simulink model "teste_linearizacao"  (R2022a)
settings: Solver=VariableStepAuto  StartTime=0.0  StopTime=10.0  RelTol=1e-3
values from neighbouring files (symbols this model uses):
  C = [0 0 1 0]    [ball_and_beam_pfc.m]
  g = 9.8    [ball_and_beam_pfc.m]    (also in nonlinear_ball_and_beam.m)
  Jv = (1/2) * mv * L^2    (= 0.058703125)    [ball_and_beam_pfc.m]    (also in nonlinear_ball_and_beam.m)
  L = 0.425    [ball_and_beam_pfc.m]    (also in nonlinear_ball_and_beam.m)
  mb = 0.064    [ball_and_beam_pfc.m]    (also in nonlinear_ball_and_beam.m)
  mv = 0.65    [ball_and_beam_pfc.m]    (also in nonlinear_ball_and_beam.m)
settings Model: Creator=Notebook_Artur  LastModifiedBy=Notebook_Artur

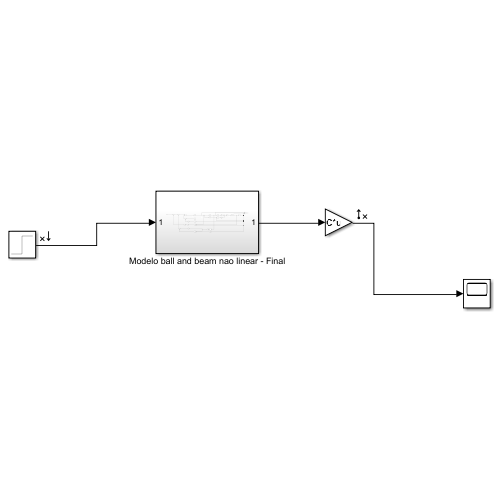
[thumbnail: Simulink's stored preview of the top-level diagram]
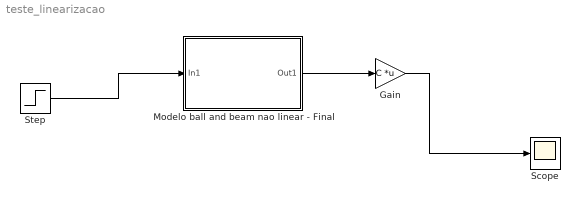
== system teste_linearizacao ==
  Gain : Gain  Gain=C  Multiplication=Matrix(K*u)
  Modelo ball and beam nao linear - Final : Subsystem
  Scope : Scope
  Step : Step  SampleTime=0
  wires:
  Step/1 -> Modelo ball and beam nao linear - Final/1(In1)
  Modelo ball and beam nao linear - Final/1(Out1) -> Gain/1
  Gain/1 -> Scope/1

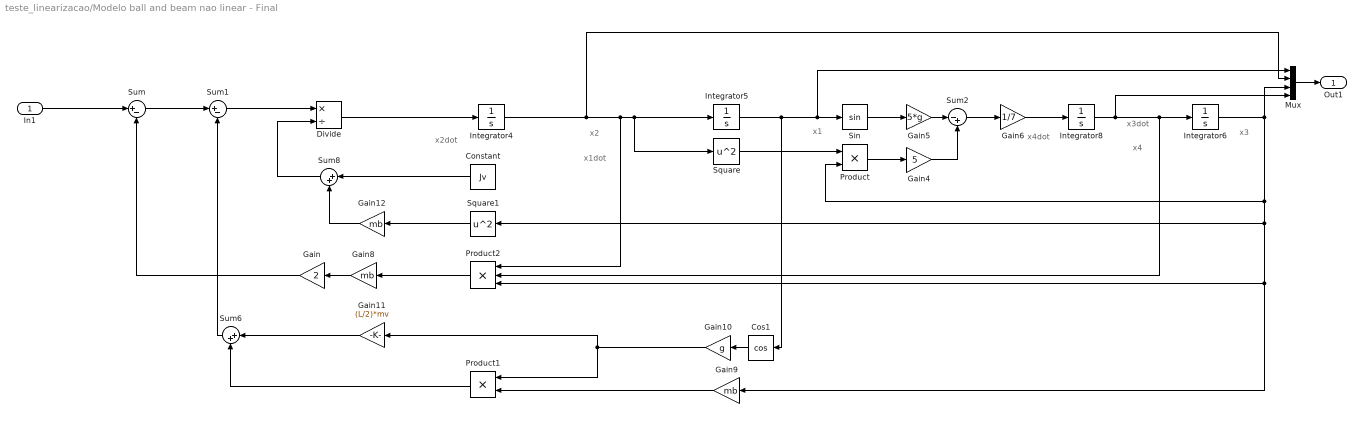
== system teste_linearizacao/Modelo ball and beam nao linear - Final ==
  note: x3
  note: x3dot
  note: x4
  note: x4dot
  note: x1
  note: x1dot
  note: x2dot
  note: x2
  In1 : Inport
  Constant : Constant  Value=Jv
  Cos1 : Trigonometry  Operator=cos
  Divide : Product  Inputs=*/
  Gain : Gain  Gain=2
  Gain10 : Gain  Gain=g
  Gain11 : Gain  Gain=(L/2)*mv
  Gain12 : Gain  Gain=mb
  Gain4 : Gain  Gain=5
  Gain5 : Gain  Gain=5*g
  Gain6 : Gain  Gain=1/7
  Gain8 : Gain  Gain=mb
  Gain9 : Gain  Gain=mb
  Integrator{4..6,8} (4 alike) : Integrator
  Mux : Mux
  Product : Product
  Product1 : Product
  Product2 : Product  Inputs=3
  Sin : Trigonometry
  Square : Math  Operator=square
  Square1 : Math  Operator=square
  Sum : Sum  Inputs=|+-
  Sum1 : Sum  Inputs=|+-
  Sum2 : Sum  Inputs=|-+
  Sum6 : Sum  Inputs=|++
  Sum8 : Sum  Inputs=|++
  Out1 : Outport
  wires:
  Integrator8/1 -> Mux/4, Product2/2, Integrator6/1
  Integrator5/1 -> Cos1/1, Sin/1, Mux/1
  Sum6/1 -> Sum1/2
  Sum2/1 -> Gain6/1
  Gain10/1 -> Product1/1, Gain11/1
  Square/1 -> Product/1
  Integrator6/1 -> Mux/3, Gain9/1, Product2/3, Square1/1, Product/2
  Gain11/1 -> Sum6/1
  Gain12/1 -> Sum8/2
  Gain6/1 -> Integrator8/1
  Gain4/1 -> Sum2/2
  Gain9/1 -> Product1/2
  Product2/1 -> Gain8/1
  Product/1 -> Gain4/1
  Square1/1 -> Gain12/1
  Product1/1 -> Sum6/2
  Constant/1 -> Sum8/1
  Mux/1 -> Out1/1
  Gain5/1 -> Sum2/1
  Sin/1 -> Gain5/1
  Gain8/1 -> Gain/1
  Sum1/1 -> Divide/1
  Sum/1 -> Sum1/1
  Gain/1 -> Sum/2
  In1/1 -> Sum/1
  Divide/1 -> Integrator4/1
  Cos1/1 -> Gain10/1
  Integrator4/1 -> Mux/2, Product2/1, Square/1, Integrator5/1
  Sum8/1 -> Divide/2
